simulink model "opti_debug"  (R2023a)
settings: Solver=FixedStepAuto  StartTime=0.0  StopTime=mdl.rt  RelTol=1e-3
values from neighbouring files (symbols this model uses):
  archived_Eul_XYZ = rst_Eul_XYZ.signals.values    [s4_run.m]    (also in step4_run_v1.m)
  archived_p_raw = rst_p_raw.signals.values    [s4_run.m]    (also in step4_run_v1.m)
  ctr = make_ext_tor_observer(rsim, mdl, ctr)    [s1_setup.m]    (also in setup_controller_with_functions.m = make_controller(); step1_setup.m; step1_setup_v1.m)
  ctr2 = ctr    [s1_setup.m]    (also in step1_setup.m; step1_setup_v1.m)
  lut = gen_lut    [s1_setup.m]    (also in thrust2voltage_lut_20230809.mat = ; thrust2voltage_lut_20230829.mat = )
  mdl = make_model(mdl,rsim)    [s1_setup.m]    (also in setup_controller_with_functions.m = make_model(flight_time); step1_setup.m; step1_setup_v1.m = make_model(flight_time,rsim))
  rbt = make_robot    [s1_setup.m]    (also in setup_controller_with_functions.m = make_robot(); step1_setup.m; step1_setup_v1.m)
  rbt2 = rbt    [s1_setup.m]    (also in step1_setup.m; step1_setup_v1.m)
  rsim = make_robot_simulation()    [setup_controller_with_functions.m]    (also in step1_setup_v1.m = make_simulation(rbt,mdl,rsim))
  sen = make_sensor(mdl,rsim)    [s1_setup.m]
  som = make_somersault(mdl, rsim)    [s1_setup.m]    (also in step1_setup.m)
  Time = logsout.LiveStreamSignals.getElement('voltage').Values.Time    [old_step3_run_controller_v3.m]    (also in post_identify_actuation_response.m = yout(:,1); post_thrust_torque_coefficients.m = yout(:,1))
  traj = make_trajectory(ctr, mdl, rsim)    [s1_setup.m]    (also in step1_setup.m)
undefined symbols (not defined in the file or in its folder): DiscIntNeverNeededParam, Discrete, Standard_Devices, UDP_Protocol
libraries: simulink x27, dspfdesign x12, robotcorelib x7, sldrtlib x7, slrealtimeloglib x1, shared6dof x1, dspsrcs4 x1, uavutilslib x1, ctrlSharedLib x1, dspmathops x1
(part 3 of 4)

== system opti_debug/State filters/Acc through derivative/Subsystem1 ==
  p_dot : Inport
  data ready : Inport  Port=2
  Add1 : Sum  Inputs=+-
  Add2 : Sum  Inputs=+-
  Add3 : Sum  Commented=on  Inputs=+-
  Add4 : Sum  Inputs=+-
  Delay : Delay  Commented=on  DelayLength=1  InitialCondition=zeros(3,1)
  Delay1 : Delay  DelayLength=1  InitialCondition=zeros(3,1)
  Digital Filter Design2 : dspfdesign/Digital Filter Design  Commented=on  mwdsp_browser_bugfix_var=off
  Digital Clock : DigitalClock  SampleTime=mdl.T_high
  Gain : Gain  Commented=on  Gain=mdl.f_high
  Gain1 : Gain  Gain=mdl.f_high
  If : If  IfExpression=u1 == 0
  If Action Subsystem : Subsystem  TreatAsAtomicUnit=on
  If Action Subsystem1 : Subsystem  TreatAsAtomicUnit=on
  Merge : Merge
  Scope : Scope  Commented=on  NumInputPorts=2
  Triggered Subsystem : Subsystem  TreatAsAtomicUnit=on
  p_dotdot : Outport
  wires:
  data ready/1 -> Triggered Subsystem/Trigger
  Triggered Subsystem/1(Out1) -> Add1/1
  Triggered Subsystem/2(Output) -> Add1/2
  Triggered Subsystem/3(Output1) -> Add2/1
  Triggered Subsystem/4(Output2) -> Add2/2
  Add1/1 -> If Action Subsystem/1(In1)
  Add2/1 -> If Action Subsystem/2(In2), If/1
  If/2 -> If Action Subsystem/Action
  If/1 -> If Action Subsystem1/Action
  If Action Subsystem1/1(Out1) -> Merge/2
  If Action Subsystem/1(Out1) -> Merge/1
  Digital Clock/1 -> Triggered Subsystem/2(In2)
  Digital Filter Design2/1 -> Delay/1, Add3/1  "p_dot_filtered"
  Delay/1 -> Add3/2
  Add3/1 -> Gain/1
  Gain/1 -> Scope/2
  Add4/1 -> Gain1/1
  Delay1/1 -> Add4/2
  p_dot/1 -> Delay1/1, Add4/1, Digital Filter Design2/1, Triggered Subsystem/1(In1)  "p_dot_filtered"
  Gain1/1 -> p_dotdot/1, Scope/1

== system opti_debug/State filters/IMU orientation/Subsystem2 ==
  euler_angles : Inport
  Add1 : Sum  Commented=on  Inputs=+-
  Add2 : Sum  Commented=on  Inputs=+-
  Digital Clock : DigitalClock  Commented=on  SampleTime=1/10000
  If : If  Commented=on  IfExpression=u1 == 0
  If Action Subsystem : Subsystem  Commented=on  TreatAsAtomicUnit=on
  If Action Subsystem1 : Subsystem  Commented=on  TreatAsAtomicUnit=on
  MATLAB Function : MATLAB Function  TreatAsAtomicUnit=on
  Merge : Merge  Commented=on
  Rotation Matrix : MATLAB Function  TreatAsAtomicUnit=on
  Rotation Matrix3 : MATLAB Function  TreatAsAtomicUnit=on
  Triggered Subsystem : Subsystem  Commented=on  TreatAsAtomicUnit=on
  Omega : Outport
  wires:
  Triggered Subsystem/1(Out1) -> Add1/1
  Triggered Subsystem/3(Output1) -> Add2/1
  Triggered Subsystem/4(Output2) -> Add2/2
  If Action Subsystem1/1(Out1) -> Merge/2
  If Action Subsystem/1(Out1) -> Merge/1
  Triggered Subsystem/2(Output) -> Add1/2
  Digital Clock/1 -> Triggered Subsystem/2(In2)
  Add2/1 -> If Action Subsystem/2(In2), If/1
  If/2 -> If Action Subsystem/Action
  If/1 -> If Action Subsystem1/Action
  Add1/1 -> If Action Subsystem/1(In1)
  euler_angles/1 -> MATLAB Function/1(Eul_in), Rotation Matrix/1(euler_angles)
  Rotation Matrix/1(R) -> Rotation Matrix3/1(R)
  Rotation Matrix3/1(w) -> Omega/1  "Vicon_omega"
  MATLAB Function/1(R_dot) -> Rotation Matrix3/2(Rdot)

== system opti_debug/State filters/Velocity through derivative/Subsystem4 ==
  In1 : Inport
  data ready : Inport  Port=2
  Add1 : Sum  Inputs=+-
  Add2 : Sum  Inputs=+-
  Digital Filter Design1 : dspfdesign/Digital Filter Design  mwdsp_browser_bugfix_var=off
  Digital Filter Design2 : dspfdesign/Digital Filter Design  Commented=on  mwdsp_browser_bugfix_var=off
  Digital Clock : DigitalClock  SampleTime=mdl.T_high
  If : If  IfExpression=u1 == 0
  If Action Subsystem : Subsystem  TreatAsAtomicUnit=on
  If Action Subsystem1 : Subsystem  TreatAsAtomicUnit=on
  Merge : Merge
  Scope : Scope  Commented=on  NumInputPorts=2
  Triggered Subsystem : Subsystem  TreatAsAtomicUnit=on
  p dot : Outport
  wires:
  In1/1 -> Triggered Subsystem/1(In1)
  data ready/1 -> Triggered Subsystem/Trigger
  Triggered Subsystem/1(Out1) -> Add1/1
  Triggered Subsystem/2(Output) -> Add1/2
  Triggered Subsystem/3(Output1) -> Add2/1
  Triggered Subsystem/4(Output2) -> Add2/2
  Add1/1 -> If Action Subsystem/1(In1)
  Add2/1 -> If Action Subsystem/2(In2), If/1
  If/2 -> If Action Subsystem/Action
  If/1 -> If Action Subsystem1/Action
  If Action Subsystem1/1(Out1) -> Merge/2
  If Action Subsystem/1(Out1) -> Merge/1
  Merge/1 -> Digital Filter Design1/1, Scope/1
  Digital Clock/1 -> Triggered Subsystem/2(In2)
  Digital Filter Design1/1 -> Scope/2, p dot/1  "p_dot_filtered"

== system opti_debug/State filters/Vicon orientation/Subsystem5 ==
  euler_angles : Inport
  data ready : Inport  Port=2
  Add1 : Sum  Inputs=+-
  Add2 : Sum  Inputs=+-
  Add3 : Sum  Inputs=+-
  Constant : Constant  Value=rsim.en
  Delay : Delay  DelayLength=1  InitialCondition=zeros(9,1)
  Digital Clock : DigitalClock  SampleTime=1/10000
  Gain : Gain  Gain=400
  If : If  IfExpression=u1 == 0
  If Action Subsystem : Subsystem  TreatAsAtomicUnit=on
  If Action Subsystem1 : Subsystem  TreatAsAtomicUnit=on
  Merge : Merge
  Rotation Matrix : MATLAB Function  TreatAsAtomicUnit=on
  Rotation Matrix2 : MATLAB Function  TreatAsAtomicUnit=on
  Rotation Matrix3 : MATLAB Function  TreatAsAtomicUnit=on
  Switch1 : Switch  Criteria=u2 > Threshold  SaturateOnIntegerOverflow=off  InputSameDT=off
  Switch2 : Switch  Criteria=u2 > Threshold  SaturateOnIntegerOverflow=off  InputSameDT=off
  Triggered Subsystem : Subsystem  TreatAsAtomicUnit=on
  R : Outport
  Rdot : Outport  Port=2
  Omega : Outport  Port=3
  wires:
  Triggered Subsystem/1(Out1) -> Add1/1
  Triggered Subsystem/3(Output1) -> Add2/1
  Triggered Subsystem/4(Output2) -> Add2/2
  If Action Subsystem1/1(Out1) -> Merge/2
  If Action Subsystem/1(Out1) -> Merge/1
  Triggered Subsystem/2(Output) -> Add1/2
  Digital Clock/1 -> Triggered Subsystem/2(In2)
  data ready/1 -> Triggered Subsystem/Trigger
  Add2/1 -> If Action Subsystem/2(In2), If/1
  If/2 -> If Action Subsystem/Action
  If/1 -> If Action Subsystem1/Action
  Add1/1 -> If Action Subsystem/1(In1)
  euler_angles/1 -> Rotation Matrix/1(euler_angles)
  Rotation Matrix/1(R) -> Triggered Subsystem/1(R), R/1, Rotation Matrix3/1(R), Rotation Matrix2/1(R), Delay/1, Add3/1
  Delay/1 -> Add3/2
  Add3/1 -> Gain/1
  Constant/1 -> Switch2/2, Switch1/2
  Gain/1 -> Switch2/1, Rotation Matrix2/2(Rdot)
  Rotation Matrix2/1(w) -> Switch1/1  "sim_omega"
  Merge/1 -> Switch2/3, Rotation Matrix3/2(Rdot)
  Rotation Matrix3/1(w) -> Switch1/3  "Vicon_omega"
  Switch1/1 -> Omega/1  "p_raw"
  Switch2/1 -> Rdot/1  "p_raw"

== system opti_debug/Control scheme/attitude and thrust controller/Yaw Controller/start ramp ==
  0.8 : Constant  Value=0.01
  2 : Constant  Value=mdl.i_delay
  Add1 : Sum
  Add2 : Sum  Inputs=+-
  Compare To Zero : simulink/Logic and Bit Operations/Compare To Zero  relop=>  OutDataTypeStr=uint8  ZeroCross=off
  Data Type Conversion : DataTypeConversion  SaturateOnIntegerOverflow=off  RndMeth=Floor
  constant : Constant
  counter : DiscreteIntegrator  gainval=1  SampleTime=-1  UpperSaturationLimit=1  LowerSaturationLimit=0  ICPrevOutput=DiscIntNeverNeededParam  ICPrevScaledInput=DiscIntNeverNeededParam
  saturation ramp : DiscreteIntegrator  gainval=5  SampleTime=-1  LimitOutput=on  UpperSaturationLimit=1  LowerSaturationLimit=-1  ICPrevOutput=DiscIntNeverNeededParam  ICPrevScaledInput=DiscIntNeverNeededParam
  Out1 : Outport
  wires:
  constant/1 -> counter/1
  2/1 -> Add1/1
  0.8/1 -> Add1/2
  counter/1 -> Add2/1
  Add1/1 -> Add2/2
  Add2/1 -> Compare To Zero/1
  Compare To Zero/1 -> Data Type Conversion/1
  saturation ramp/1 -> Out1/1
  Data Type Conversion/1 -> saturation ramp/1

== system opti_debug/Control scheme/observer/Rotaion/filtered derivative ==
  In1 : Inport
  att_s : Gain  Gain=mdl.f1
  filtered derivative : simulink/Discrete/Transfer Fcn Lead or Lag  PoleZ=mdl.zf1  ZeroZ=1  ICPrevOutput=0.0  ICPrevInput=0.0  DoSatur=off
  low pass3 : DiscreteTransferFcn  Numerator=mdl.vlp.n  Denominator=mdl.vlp.d
  Out1 : Outport
  wires:
  filtered derivative/1 -> low pass3/1
  att_s/1 -> filtered derivative/1
  In1/1 -> att_s/1
  low pass3/1 -> Out1/1

== system opti_debug/Control scheme/observer/lateral observer/saturation ==
  In1 : Inport
  MinMax2 : MinMax  Inputs=2
  MinMax3 : MinMax  Function=max  Inputs=2
  lw1 : Constant  Value=-mdl.fd_lim
  up1 : Constant  Value=mdl.fd_lim
  Out1 : Outport
  wires:
  In1/1 -> MinMax2/2
  up1/1 -> MinMax2/1
  lw1/1 -> MinMax3/1
  MinMax2/1 -> MinMax3/2
  MinMax3/1 -> Out1/1

== system opti_debug/Signal generater/signal generator1/Bias_Signal/AveragedBias ==
  note: To avoid having signal "jump",
      | we want SMOOTH transitions
      | in frequency (i.e., a weighted sum
      | of current freq and freq some delta t ago)
  note: time constant = 0.002sec
  In1 : Inport
  Discrete Transfer Fcn : DiscreteTransferFcn  Commented=through  Numerator=[0.05]  Denominator=[1 -.95]
  Out1 : Outport
  wires:
  In1/1 -> Discrete Transfer Fcn/1
  Discrete Transfer Fcn/1 -> Out1/1

== system opti_debug/Signal generater/signal generator1/Bias_Signal/SIgnalForRamp_binary ==
  note: Should output 1 or -1,
      | so signal ramps UP to 1
      | or DOWN to 0.
  In1 : Inport
  Add : Sum  Inputs=+-
  Compare To Zero : simulink/Logic and Bit Operations/Compare To Zero  relop=>  OutDataTypeStr=uint8  ZeroCross=off
  Constant : Constant
  Data Type Conversion : DataTypeConversion  OutDataTypeStr=double  SaturateOnIntegerOverflow=off  RndMeth=Floor
  Gain : Gain  Gain=2
  Out1 : Outport
  wires:
  In1/1 -> Compare To Zero/1
  Compare To Zero/1 -> Data Type Conversion/1
  Gain/1 -> Add/1
  Constant/1 -> Add/2
  Add/1 -> Out1/1
  Data Type Conversion/1 -> Gain/1

== system opti_debug/Signal generater/signal generator1/Drive_Signal1/AveragedAmp_filtered ==
  note: To avoid having signal "jump",
      | we want SMOOTH transitions
      | in frequency (i.e., a weighted sum
      | of current freq and freq some delta t ago)
  note: time constant 0.002sec
      | for 10kHz samping
  In1 : Inport
  Discrete Transfer Fcn : DiscreteTransferFcn  Commented=through  Numerator=[0.05]  Denominator=[1 -.95]
  Out1 : Outport
  wires:
  In1/1 -> Discrete Transfer Fcn/1
  Discrete Transfer Fcn/1 -> Out1/1

== system opti_debug/Signal generater/signal generator1/Drive_Signal1/AveragedOffset_filtered ==
  note: To avoid having signal "jump",
      | we want SMOOTH transitions
      | in frequency (i.e., a weighted sum
      | of current freq and freq some delta t ago)
  note: c
  note: time constant 0.02sec
      | for 10kHz samping
  In1 : Inport
  Discrete Transfer Fcn : DiscreteTransferFcn  Commented=through  Numerator=[0.05]  Denominator=[1 -.95]
  Out1 : Outport
  wires:
  In1/1 -> Discrete Transfer Fcn/1
  Discrete Transfer Fcn/1 -> Out1/1

== system opti_debug/Signal generater/signal generator1/Drive_Signal1/AveragedTau_filtered ==
  note: To avoid having signal "jump",
      | we want SMOOTH transitions
      | in frequency (i.e., a weighted sum
      | of current freq and freq some delta t ago)
  note: time constant 0.002sec
      | for 10kHz samping
  In1 : Inport
  Discrete Transfer Fcn : DiscreteTransferFcn  Numerator=[0.05]  Denominator=[1, -0.95]
  Out1 : Outport
  wires:
  In1/1 -> Discrete Transfer Fcn/1
  Discrete Transfer Fcn/1 -> Out1/1

== system opti_debug/Signal generater/signal generator1/Drive_Signal1/SignalForRamp_binary ==
  note: Should output 1 or -1,
      | so signal ramps UP to 1
      | or DOWN to 0.
  In1 : Inport
  Add : Sum  Inputs=+-
  Compare To Zero : simulink/Logic and Bit Operations/Compare To Zero  relop=>  OutDataTypeStr=uint8  ZeroCross=off
  Constant : Constant
  Data Type Conversion : DataTypeConversion  OutDataTypeStr=double  SaturateOnIntegerOverflow=off  RndMeth=Floor
  Gain : Gain  Gain=2
  Out1 : Outport
  wires:
  In1/1 -> Compare To Zero/1
  Compare To Zero/1 -> Data Type Conversion/1
  Gain/1 -> Add/1
  Constant/1 -> Add/2
  Add/1 -> Out1/1
  Data Type Conversion/1 -> Gain/1

== system opti_debug/Signal generater/signal generator1/Drive_Signal1/SignalForSin_binary ==
  note: We want this to stay "high" for 1
      | second after the actual "enable"
      | is turned off...
  In1 : Inport
  Compare To Zero : simulink/Logic and Bit Operations/Compare To Zero  relop=>  OutDataTypeStr=uint8  ZeroCross=off
  Data Type Conversion : DataTypeConversion  OutDataTypeStr=double  SaturateOnIntegerOverflow=off  RndMeth=Floor
  Out1 : Outport
  wires:
  In1/1 -> Compare To Zero/1
  Compare To Zero/1 -> Data Type Conversion/1
  Data Type Conversion/1 -> Out1/1

== system opti_debug/Signal generater/signal generator1/Drive_Signal1/Subsystem ==
  note: positive value pushes the left wing forward
  split cycle mu : Inport
  In2 : Inport  Port=2
  1-mu : Sum  Inputs=+-
  2f : Gain  Gain=2
  2nd harmonic : Trigonometry  OutputSignalType=real
  2pi : Gain  Gain=2*pi
  Abs1 : Abs  SaturateOnIntegerOverflow=off
  Add : Sum
  Constant : Constant
  combined sines : Sum
  deg to rad : Gain  Gain=pi/180
  f : Gain  Gain=-1
  first harmonic : Trigonometry  OutputSignalType=real
  omega*t : DiscreteIntegrator  SampleTime=-1  ICPrevOutput=DiscIntNeverNeededParam  ICPrevScaledInput=DiscIntNeverNeededParam
  phase offset : Constant  Value=0
  signal with gain1 : Product  RndMeth=Zero
  signal with gain2 : Product  RndMeth=Zero
  split cycle signal : Outport
  wires:
  2f/1 -> 2nd harmonic/1
  first harmonic/1 -> signal with gain1/2
  Constant/1 -> 1-mu/1
  split cycle mu/1 -> f/1, Abs1/1
  1-mu/1 -> signal with gain1/1
  2nd harmonic/1 -> signal with gain2/2
  signal with gain1/1 -> combined sines/1
  signal with gain2/1 -> combined sines/2
  combined sines/1 -> split cycle signal/1
  f/1 -> signal with gain2/1
  Abs1/1 -> 1-mu/2
  In2/1 -> 2pi/1
  2pi/1 -> omega*t/1
  omega*t/1 -> Add/2
  Add/1 -> first harmonic/1, 2f/1
  phase offset/1 -> deg to rad/1
  deg to rad/1 -> Add/1

== system opti_debug/Signal generater/signal generator1/Drive_Signal2/AveragedAmp_filtered ==
  note: To avoid having signal "jump",
      | we want SMOOTH transitions
      | in frequency (i.e., a weighted sum
      | of current freq and freq some delta t ago)
  note: time constant 0.002sec
      | for 10kHz samping
  In1 : Inport
  Discrete Transfer Fcn : DiscreteTransferFcn  Numerator=[0.05]  Denominator=[1 -.95]
  Out1 : Outport
  wires:
  In1/1 -> Discrete Transfer Fcn/1
  Discrete Transfer Fcn/1 -> Out1/1

== system opti_debug/Signal generater/signal generator1/Drive_Signal2/AveragedOffset_filtered ==
  note: To avoid having signal "jump",
      | we want SMOOTH transitions
      | in frequency (i.e., a weighted sum
      | of current freq and freq some delta t ago)
  note: c
  note: time constant 0.02sec
      | for 10kHz samping
  In1 : Inport
  Discrete Transfer Fcn : DiscreteTransferFcn  Numerator=[0.05]  Denominator=[1 -.95]
  Out1 : Outport
  wires:
  In1/1 -> Discrete Transfer Fcn/1
  Discrete Transfer Fcn/1 -> Out1/1

== system opti_debug/Signal generater/signal generator1/Drive_Signal2/AveragedTau_filtered ==
  note: To avoid having signal "jump",
      | we want SMOOTH transitions
      | in frequency (i.e., a weighted sum
      | of current freq and freq some delta t ago)
  note: time constant 0.002sec
      | for 10kHz samping
  In1 : Inport
  Discrete Transfer Fcn : DiscreteTransferFcn  Numerator=[0.05]  Denominator=[1, -0.95]
  Out1 : Outport
  wires:
  In1/1 -> Discrete Transfer Fcn/1
  Discrete Transfer Fcn/1 -> Out1/1

== system opti_debug/Signal generater/signal generator1/Drive_Signal2/SignalForRamp_binary ==
  note: Should output 1 or -1,
      | so signal ramps UP to 1
      | or DOWN to 0.
  In1 : Inport
  Add : Sum  Inputs=+-
  Compare To Zero : simulink/Logic and Bit Operations/Compare To Zero  relop=>  OutDataTypeStr=uint8  ZeroCross=off
  Constant : Constant
  Data Type Conversion : DataTypeConversion  OutDataTypeStr=double  SaturateOnIntegerOverflow=off  RndMeth=Floor
  Gain : Gain  Gain=2
  Out1 : Outport
  wires:
  In1/1 -> Compare To Zero/1
  Compare To Zero/1 -> Data Type Conversion/1
  Gain/1 -> Add/1
  Constant/1 -> Add/2
  Add/1 -> Out1/1
  Data Type Conversion/1 -> Gain/1

== system opti_debug/Signal generater/signal generator1/Drive_Signal2/SignalForSin_binary ==
  note: We want this to stay "high" for 1
      | second after the actual "enable"
      | is turned off...
  In1 : Inport
  Compare To Zero : simulink/Logic and Bit Operations/Compare To Zero  relop=>  OutDataTypeStr=uint8  ZeroCross=off
  Data Type Conversion : DataTypeConversion  OutDataTypeStr=double  SaturateOnIntegerOverflow=off  RndMeth=Floor
  Out1 : Outport
  wires:
  In1/1 -> Compare To Zero/1
  Compare To Zero/1 -> Data Type Conversion/1
  Data Type Conversion/1 -> Out1/1

== system opti_debug/Signal generater/signal generator1/Drive_Signal2/Subsystem ==
  note: positive value pushes the left wing forward
  split cycle mu : Inport
  In2 : Inport  Port=2
  1-mu : Sum  Inputs=+-
  2f : Gain  Gain=2
  2nd harmonic : Trigonometry  OutputSignalType=real
  2pi : Gain  Gain=2*pi
  Abs1 : Abs  SaturateOnIntegerOverflow=off
  Add : Sum
  Constant : Constant
  combined sines : Sum
  deg to rad : Gain  Gain=pi/180
  f : Gain  Gain=-1
  first harmonic : Trigonometry  OutputSignalType=real
  omega*t : DiscreteIntegrator  SampleTime=-1  ICPrevOutput=DiscIntNeverNeededParam  ICPrevScaledInput=DiscIntNeverNeededParam
  phase offset : Constant  Value=0
  signal with gain1 : Product  RndMeth=Zero
  signal with gain2 : Product  RndMeth=Zero
  split cycle signal : Outport
  wires:
  2f/1 -> 2nd harmonic/1
  first harmonic/1 -> signal with gain1/2
  Constant/1 -> 1-mu/1
  split cycle mu/1 -> f/1, Abs1/1
  1-mu/1 -> signal with gain1/1
  2nd harmonic/1 -> signal with gain2/2
  signal with gain1/1 -> combined sines/1
  signal with gain2/1 -> combined sines/2
  combined sines/1 -> split cycle signal/1
  f/1 -> signal with gain2/1
  Abs1/1 -> 1-mu/2
  In2/1 -> 2pi/1
  2pi/1 -> omega*t/1
  omega*t/1 -> Add/2
  Add/1 -> first harmonic/1, 2f/1
  phase offset/1 -> deg to rad/1
  deg to rad/1 -> Add/1

== system opti_debug/Signal generater/signal generator1/Drive_Signal3/AveragedAmp_filtered ==
  note: To avoid having signal "jump",
      | we want SMOOTH transitions
      | in frequency (i.e., a weighted sum
      | of current freq and freq some delta t ago)
  note: time constant 0.002sec
      | for 10kHz samping
  In1 : Inport
  Discrete Transfer Fcn : DiscreteTransferFcn  Numerator=[0.05]  Denominator=[1 -.95]
  Out1 : Outport
  wires:
  In1/1 -> Discrete Transfer Fcn/1
  Discrete Transfer Fcn/1 -> Out1/1

== system opti_debug/Signal generater/signal generator1/Drive_Signal3/AveragedOffset_filtered ==
  note: To avoid having signal "jump",
      | we want SMOOTH transitions
      | in frequency (i.e., a weighted sum
      | of current freq and freq some delta t ago)
  note: c
  note: time constant 0.02sec
      | for 10kHz samping
  In1 : Inport
  Discrete Transfer Fcn : DiscreteTransferFcn  Numerator=[0.05]  Denominator=[1 -.95]
  Out1 : Outport
  wires:
  In1/1 -> Discrete Transfer Fcn/1
  Discrete Transfer Fcn/1 -> Out1/1

== system opti_debug/Signal generater/signal generator1/Drive_Signal3/AveragedTau_filtered ==
  note: To avoid having signal "jump",
      | we want SMOOTH transitions
      | in frequency (i.e., a weighted sum
      | of current freq and freq some delta t ago)
  note: time constant 0.002sec
      | for 10kHz samping
  In1 : Inport
  Discrete Transfer Fcn : DiscreteTransferFcn  Numerator=[0.05]  Denominator=[1 -.95]
  Out1 : Outport
  wires:
  In1/1 -> Discrete Transfer Fcn/1
  Discrete Transfer Fcn/1 -> Out1/1

== system opti_debug/Signal generater/signal generator1/Drive_Signal3/SignalForRamp_binary ==
  note: Should output 1 or -1,
      | so signal ramps UP to 1
      | or DOWN to 0.
  In1 : Inport
  Add : Sum  Inputs=+-
  Compare To Zero : simulink/Logic and Bit Operations/Compare To Zero  relop=>  OutDataTypeStr=uint8  ZeroCross=off
  Constant : Constant
  Data Type Conversion : DataTypeConversion  OutDataTypeStr=double  SaturateOnIntegerOverflow=off  RndMeth=Floor
  Gain : Gain  Gain=2
  Out1 : Outport
  wires:
  In1/1 -> Compare To Zero/1
  Compare To Zero/1 -> Data Type Conversion/1
  Gain/1 -> Add/1
  Constant/1 -> Add/2
  Add/1 -> Out1/1
  Data Type Conversion/1 -> Gain/1

== system opti_debug/Signal generater/signal generator1/Drive_Signal3/SignalForSin_binary ==
  note: We want this to stay "high" for 1
      | second after the actual "enable"
      | is turned off...
  In1 : Inport
  Compare To Zero : simulink/Logic and Bit Operations/Compare To Zero  relop=>  OutDataTypeStr=uint8  ZeroCross=off
  Data Type Conversion : DataTypeConversion  OutDataTypeStr=double  SaturateOnIntegerOverflow=off  RndMeth=Floor
  Out1 : Outport
  wires:
  In1/1 -> Compare To Zero/1
  Compare To Zero/1 -> Data Type Conversion/1
  Data Type Conversion/1 -> Out1/1

== system opti_debug/Signal generater/signal generator1/Drive_Signal3/Subsystem ==
  split cycle mu : Inport
  In2 : Inport  Port=2
  1-mu : Sum  Inputs=+-
  2f : Gain  Gain=2
  2nd harmonic : Trigonometry  OutputSignalType=real
  2pi : Gain  Gain=2*pi
  Abs1 : Abs  SaturateOnIntegerOverflow=off
  Constant : Constant
  SmoothClock : DiscreteIntegrator  SampleTime=-1  ICPrevOutput=DiscIntNeverNeededParam  ICPrevScaledInput=DiscIntNeverNeededParam
  combined sines : Sum
  f : Gain
  first harmonic : Trigonometry  OutputSignalType=real
  signal with gain1 : Product  RndMeth=Zero
  signal with gain2 : Product  RndMeth=Zero
  split cycle signal : Outport
  wires:
  SmoothClock/1 -> first harmonic/1, 2f/1
  2f/1 -> 2nd harmonic/1
  2pi/1 -> SmoothClock/1
  first harmonic/1 -> signal with gain1/2
  Constant/1 -> 1-mu/1
  split cycle mu/1 -> f/1, Abs1/1
  1-mu/1 -> signal with gain1/1
  2nd harmonic/1 -> signal with gain2/2
  signal with gain1/1 -> combined sines/1
  signal with gain2/1 -> combined sines/2
  combined sines/1 -> split cycle signal/1
  In2/1 -> 2pi/1
  f/1 -> signal with gain2/1
  Abs1/1 -> 1-mu/2

== system opti_debug/Signal generater/signal generator1/Drive_Signal4/AveragedAmp_filtered ==
  note: To avoid having signal "jump",
      | we want SMOOTH transitions
      | in frequency (i.e., a weighted sum
      | of current freq and freq some delta t ago)
  note: time constant 0.002sec
      | for 10kHz samping
  In1 : Inport
  Discrete Transfer Fcn : DiscreteTransferFcn  Commented=through  Numerator=[0.05]  Denominator=[1 -.95]
  Out1 : Outport
  wires:
  In1/1 -> Discrete Transfer Fcn/1
  Discrete Transfer Fcn/1 -> Out1/1

== system opti_debug/Signal generater/signal generator1/Drive_Signal4/AveragedOffset_filtered ==
  note: To avoid having signal "jump",
      | we want SMOOTH transitions
      | in frequency (i.e., a weighted sum
      | of current freq and freq some delta t ago)
  note: c
  note: time constant 0.02sec
      | for 10kHz samping
  In1 : Inport
  Discrete Transfer Fcn : DiscreteTransferFcn  Commented=through  Numerator=[0.05]  Denominator=[1 -.95]
  Out1 : Outport
  wires:
  In1/1 -> Discrete Transfer Fcn/1
  Discrete Transfer Fcn/1 -> Out1/1

== system opti_debug/Signal generater/signal generator1/Drive_Signal4/AveragedTau_filtered ==
  note: To avoid having signal "jump",
      | we want SMOOTH transitions
      | in frequency (i.e., a weighted sum
      | of current freq and freq some delta t ago)
  note: time constant 0.002sec
      | for 10kHz samping
  In1 : Inport
  Discrete Transfer Fcn : DiscreteTransferFcn  Numerator=[0.05]  Denominator=[1, -0.95]
  Out1 : Outport
  wires:
  In1/1 -> Discrete Transfer Fcn/1
  Discrete Transfer Fcn/1 -> Out1/1

== system opti_debug/Signal generater/signal generator1/Drive_Signal4/SignalForRamp_binary ==
  note: Should output 1 or -1,
      | so signal ramps UP to 1
      | or DOWN to 0.
  In1 : Inport
  Add : Sum  Inputs=+-
  Compare To Zero : simulink/Logic and Bit Operations/Compare To Zero  relop=>  OutDataTypeStr=uint8  ZeroCross=off
  Constant : Constant
  Data Type Conversion : DataTypeConversion  OutDataTypeStr=double  SaturateOnIntegerOverflow=off  RndMeth=Floor
  Gain : Gain  Gain=2
  Out1 : Outport
  wires:
  In1/1 -> Compare To Zero/1
  Compare To Zero/1 -> Data Type Conversion/1
  Gain/1 -> Add/1
  Constant/1 -> Add/2
  Add/1 -> Out1/1
  Data Type Conversion/1 -> Gain/1

== system opti_debug/Signal generater/signal generator1/Drive_Signal4/SignalForSin_binary ==
  note: We want this to stay "high" for 1
      | second after the actual "enable"
      | is turned off...
  In1 : Inport
  Compare To Zero : simulink/Logic and Bit Operations/Compare To Zero  relop=>  OutDataTypeStr=uint8  ZeroCross=off
  Data Type Conversion : DataTypeConversion  OutDataTypeStr=double  SaturateOnIntegerOverflow=off  RndMeth=Floor
  Out1 : Outport
  wires:
  In1/1 -> Compare To Zero/1
  Compare To Zero/1 -> Data Type Conversion/1
  Data Type Conversion/1 -> Out1/1

== system opti_debug/Signal generater/signal generator1/Drive_Signal4/Subsystem ==
  note: positive value pushes the left wing forward
  split cycle mu : Inport
  In2 : Inport  Port=2
  1-mu : Sum  Inputs=+-
  2f : Gain  Gain=2
  2nd harmonic : Trigonometry  OutputSignalType=real
  2pi : Gain  Gain=2*pi
  Abs1 : Abs  SaturateOnIntegerOverflow=off
  Add : Sum
  Constant : Constant
  combined sines : Sum
  deg to rad : Gain  Gain=pi/180
  f : Gain  Gain=-1
  first harmonic : Trigonometry  OutputSignalType=real
  omega*t : DiscreteIntegrator  SampleTime=-1  ICPrevOutput=DiscIntNeverNeededParam  ICPrevScaledInput=DiscIntNeverNeededParam
  phase offset : Constant  Value=0
  signal with gain1 : Product  RndMeth=Zero
  signal with gain2 : Product  RndMeth=Zero
  split cycle signal : Outport
  wires:
  2f/1 -> 2nd harmonic/1
  first harmonic/1 -> signal with gain1/2
  Constant/1 -> 1-mu/1
  split cycle mu/1 -> f/1, Abs1/1
  1-mu/1 -> signal with gain1/1
  2nd harmonic/1 -> signal with gain2/2
  signal with gain1/1 -> combined sines/1
  signal with gain2/1 -> combined sines/2
  combined sines/1 -> split cycle signal/1
  f/1 -> signal with gain2/1
  Abs1/1 -> 1-mu/2
  In2/1 -> 2pi/1
  2pi/1 -> omega*t/1
  omega*t/1 -> Add/2
  Add/1 -> first harmonic/1, 2f/1
  phase offset/1 -> deg to rad/1
  deg to rad/1 -> Add/1

== system opti_debug/Signal generater/signal generator1/signal generator 1/SignalForRamp_binary ==
  note: Should output 1 or -1,
      | so signal ramps UP to 1
      | or DOWN to 0.
  EnableSignal : Inport
  Add : Sum  Inputs=+-
  Compare To Zero : simulink/Logic and Bit Operations/Compare To Zero  relop=>  OutDataTypeStr=uint8  ZeroCross=off
  Constant : Constant
  Data Type Conversion : DataTypeConversion  OutDataTypeStr=double  SaturateOnIntegerOverflow=off  RndMeth=Floor
  Gain : Gain  Gain=2
  Out1 : Outport
  wires:
  EnableSignal/1 -> Compare To Zero/1
  Compare To Zero/1 -> Data Type Conversion/1
  Gain/1 -> Add/1
  Constant/1 -> Add/2
  Add/1 -> Out1/1
  Data Type Conversion/1 -> Gain/1

== system opti_debug/Signal generater/signal generator1/signal generator 1/SignalSaturationLimit4 ==
  Max : Inport
  SignalRaw : Inport  Port=2
  MaxOf : MinMax  Function=max  Inputs=2
  MinOf : MinMax  Inputs=2
  ground : Constant
  SignalSatd : Outport
  wires:
  SignalRaw/1 -> MinOf/2
  MinOf/1 -> MaxOf/1
  MaxOf/1 -> SignalSatd/1
  Max/1 -> MinOf/1
  ground/1 -> MaxOf/2

== system opti_debug/Signal generater/signal generator1/signal generator 1/get max voltage ==
  note: time constant = 0.002sec
  QuasiEnable : Inport
  max voltage : Inport  Port=2
  Product : Product  RndMeth=Zero
  SIgnalForRamp_binary : Subsystem
  SaturatingRamp : DiscreteIntegrator  gainval=1000  SampleTime=-1  LimitOutput=on  UpperSaturationLimit=1  LowerSaturationLimit=0  ICPrevOutput=DiscIntNeverNeededParam  ICPrevScaledInput=DiscIntNeverNeededParam
  max signa; : Outport
  wires:
  Product/1 -> max signa;/1
  max voltage/1 -> Product/2
  QuasiEnable/1 -> SIgnalForRamp_binary/1(In1)
  SIgnalForRamp_binary/1(Out1) -> SaturatingRamp/1
  SaturatingRamp/1 -> Product/1

== system opti_debug/Signal generater/signal generator1/signal generator 1/original sine wave ==
  In1 : Inport
  In2 : Inport  Port=2
  new_amplitude : Inport  Port=3
  2pi : Gain  Gain=2*pi
  Add1 : Sum
  Add2 : Sum
  Gain1 : Gain  Gain=-1
  Subsystem : Subsystem
  first harmonic : Trigonometry  Operator=cos  OutputSignalType=real
  omega*t : DiscreteIntegrator  SampleTime=-1  ICPrevOutput=DiscIntNeverNeededParam  ICPrevScaledInput=DiscIntNeverNeededParam
  signal with gain1 : Product  RndMeth=Zero
  Out1 : Outport
  wires:
  signal with gain1/1 -> Add2/1
  first harmonic/1 -> Gain1/1
  omega*t/1 -> Add1/2
  Subsystem/1(output) -> signal with gain1/2, Add2/2
  In2/1 -> 2pi/1
  Add1/1 -> first harmonic/1
  Gain1/1 -> Subsystem/1(cos wave), signal with gain1/1
  2pi/1 -> omega*t/1
  In1/1 -> Add1/1
  Add2/1 -> Out1/1
  new_amplitude/1 -> Subsystem/2(new_amplitude)

== system opti_debug/Signal generater/signal generator1/signal generator 1/square root of sine wave ==
  phase : Inport
  frequency : Inport  Port=2
  half amplitude : Inport  Port=3
  2pi1 : Gain  Gain=2*pi
  Add : Sum
  Add3 : Sum
  Constant : Constant
  Gain : Gain  Gain=2
  Gain2 : Gain  Gain=1/sqrt(2)
  Sqrt : Sqrt
  Subsystem1 : Subsystem
  first harmonic1 : Trigonometry  Operator=cos  OutputSignalType=real
  omega*t1 : DiscreteIntegrator  SampleTime=-1  ICPrevOutput=DiscIntNeverNeededParam  ICPrevScaledInput=DiscIntNeverNeededParam
  signal with gain2 : Product  RndMeth=Zero
  Out1 : Outport
  wires:
  frequency/1 -> 2pi1/1
  Sqrt/1 -> Subsystem1/1(cos wave), signal with gain2/1
  Gain/1 -> Subsystem1/2(new_amplitude)
  Subsystem1/1(output) -> signal with gain2/2
  omega*t1/1 -> Add3/2
  first harmonic1/1 -> Add/1
  Constant/1 -> Add/2
  2pi1/1 -> omega*t1/1
  signal with gain2/1 -> Gain2/1
  Add/1 -> Sqrt/1
  Add3/1 -> first harmonic1/1
  half amplitude/1 -> Gain/1
  phase/1 -> Add3/1
  Gain2/1 -> Out1/1

== system opti_debug/Signal generater/signal generator1/signal generator 2/SignalForRamp_binary ==
  note: Should output 1 or -1,
      | so signal ramps UP to 1
      | or DOWN to 0.
  EnableSignal : Inport
  Add : Sum  Inputs=+-
  Compare To Zero : simulink/Logic and Bit Operations/Compare To Zero  relop=>  OutDataTypeStr=uint8  ZeroCross=off
  Constant : Constant
  Data Type Conversion : DataTypeConversion  OutDataTypeStr=double  SaturateOnIntegerOverflow=off  RndMeth=Floor
  Gain : Gain  Gain=2
  Out1 : Outport
  wires:
  EnableSignal/1 -> Compare To Zero/1
  Compare To Zero/1 -> Data Type Conversion/1
  Gain/1 -> Add/1
  Constant/1 -> Add/2
  Add/1 -> Out1/1
  Data Type Conversion/1 -> Gain/1

== system opti_debug/Signal generater/signal generator1/signal generator 2/SignalSaturationLimit4 ==
  Max : Inport
  SignalRaw : Inport  Port=2
  MaxOf : MinMax  Function=max  Inputs=2
  MinOf : MinMax  Inputs=2
  ground : Constant
  SignalSatd : Outport
  wires:
  SignalRaw/1 -> MinOf/2
  MinOf/1 -> MaxOf/1
  MaxOf/1 -> SignalSatd/1
  Max/1 -> MinOf/1
  ground/1 -> MaxOf/2

== system opti_debug/Signal generater/signal generator1/signal generator 2/Subsystem ==
  cos wave : Inport
  new_amplitude : Inport  Port=2
  Delay : Delay  DelayLength=1  InitialCondition=0
  Delay1 : Delay  InitialCondition=[0,0]
  Delay2 : Delay  DelayLength=1  InitialCondition=0
  MATLAB Function : MATLAB Function  TreatAsAtomicUnit=on  SystemSampleTime=mdl.T_high
  output : Outport
  wires:
  cos wave/1 -> Delay1/1, Delay/1, MATLAB Function/1(u1)
  MATLAB Function/1(output) -> output/1, Delay2/1
  Delay/1 -> MATLAB Function/2(u2)
  Delay2/1 -> MATLAB Function/5(old_amplitude)
  Delay1/1 -> MATLAB Function/3(u3)
  new_amplitude/1 -> MATLAB Function/4(new_amplitude)

== system opti_debug/Signal generater/signal generator1/signal generator 2/get max voltage ==
  note: time constant = 0.002sec
  QuasiEnable : Inport
  max voltage : Inport  Port=2
  Product : Product  RndMeth=Zero
  SIgnalForRamp_binary : Subsystem
  SaturatingRamp : DiscreteIntegrator  gainval=1000  SampleTime=-1  LimitOutput=on  UpperSaturationLimit=1  LowerSaturationLimit=0  ICPrevOutput=DiscIntNeverNeededParam  ICPrevScaledInput=DiscIntNeverNeededParam
  max signa; : Outport
  wires:
  Product/1 -> max signa;/1
  max voltage/1 -> Product/2
  QuasiEnable/1 -> SIgnalForRamp_binary/1(In1)
  SIgnalForRamp_binary/1(Out1) -> SaturatingRamp/1
  SaturatingRamp/1 -> Product/1

== system opti_debug/Signal generater/signal generator1/signal generator 2/square root of sine wave ==
  phase : Inport
  frequency : Inport  Port=2
  half amplitude : Inport  Port=3
  2pi1 : Gain  Gain=2*pi
  Add : Sum
  Add3 : Sum
  Constant : Constant
  Gain : Gain  Gain=2
  Gain2 : Gain  Gain=1/sqrt(2)
  Sqrt : Sqrt
  Subsystem1 : Subsystem
  first harmonic1 : Trigonometry  Operator=cos  OutputSignalType=real
  omega*t1 : DiscreteIntegrator  SampleTime=-1  ICPrevOutput=DiscIntNeverNeededParam  ICPrevScaledInput=DiscIntNeverNeededParam
  signal with gain2 : Product  RndMeth=Zero
  Out1 : Outport
  wires:
  frequency/1 -> 2pi1/1
  Sqrt/1 -> Subsystem1/1(cos wave), signal with gain2/1
  Gain/1 -> Subsystem1/2(new_amplitude)
  Subsystem1/1(output) -> signal with gain2/2
  omega*t1/1 -> Add3/2
  first harmonic1/1 -> Add/1
  Constant/1 -> Add/2
  2pi1/1 -> omega*t1/1
  signal with gain2/1 -> Gain2/1
  Add/1 -> Sqrt/1
  Add3/1 -> first harmonic1/1
  half amplitude/1 -> Gain/1
  phase/1 -> Add3/1
  Gain2/1 -> Out1/1

== system opti_debug/Signal generater/signal generator1/signal generator 3/SignalForRamp_binary ==
  note: Should output 1 or -1,
      | so signal ramps UP to 1
      | or DOWN to 0.
  EnableSignal : Inport
  Add : Sum  Inputs=+-
  Compare To Zero : simulink/Logic and Bit Operations/Compare To Zero  relop=>  OutDataTypeStr=uint8  ZeroCross=off
  Constant : Constant
  Data Type Conversion : DataTypeConversion  OutDataTypeStr=double  SaturateOnIntegerOverflow=off  RndMeth=Floor
  Gain : Gain  Gain=2
  Out1 : Outport
  wires:
  EnableSignal/1 -> Compare To Zero/1
  Compare To Zero/1 -> Data Type Conversion/1
  Gain/1 -> Add/1
  Constant/1 -> Add/2
  Add/1 -> Out1/1
  Data Type Conversion/1 -> Gain/1

== system opti_debug/Signal generater/signal generator1/signal generator 3/SignalSaturationLimit4 ==
  Max : Inport
  SignalRaw : Inport  Port=2
  MaxOf : MinMax  Function=max  Inputs=2
  MinOf : MinMax  Inputs=2
  ground : Constant
  SignalSatd : Outport
  wires:
  SignalRaw/1 -> MinOf/2
  MinOf/1 -> MaxOf/1
  MaxOf/1 -> SignalSatd/1
  Max/1 -> MinOf/1
  ground/1 -> MaxOf/2

== system opti_debug/Signal generater/signal generator1/signal generator 3/Subsystem ==
  cos wave : Inport
  new_amplitude : Inport  Port=2
  Delay : Delay  DelayLength=1  InitialCondition=0
  Delay1 : Delay  InitialCondition=[0,0]
  Delay2 : Delay  DelayLength=1  InitialCondition=0
  MATLAB Function : MATLAB Function  TreatAsAtomicUnit=on  SystemSampleTime=mdl.T_high
  output : Outport
  wires:
  cos wave/1 -> Delay1/1, Delay/1, MATLAB Function/1(u1)
  MATLAB Function/1(output) -> output/1, Delay2/1
  Delay/1 -> MATLAB Function/2(u2)
  Delay2/1 -> MATLAB Function/5(old_amplitude)
  Delay1/1 -> MATLAB Function/3(u3)
  new_amplitude/1 -> MATLAB Function/4(new_amplitude)

== system opti_debug/Signal generater/signal generator1/signal generator 3/get max voltage ==
  note: time constant = 0.002sec
  QuasiEnable : Inport
  max voltage : Inport  Port=2
  Product : Product  RndMeth=Zero
  SIgnalForRamp_binary : Subsystem
  SaturatingRamp : DiscreteIntegrator  gainval=1000  SampleTime=-1  LimitOutput=on  UpperSaturationLimit=1  LowerSaturationLimit=0  ICPrevOutput=DiscIntNeverNeededParam  ICPrevScaledInput=DiscIntNeverNeededParam
  max signa; : Outport
  wires:
  Product/1 -> max signa;/1
  max voltage/1 -> Product/2
  QuasiEnable/1 -> SIgnalForRamp_binary/1(In1)
  SIgnalForRamp_binary/1(Out1) -> SaturatingRamp/1
  SaturatingRamp/1 -> Product/1

== system opti_debug/Signal generater/signal generator1/signal generator 3/square root of sine wave ==
  phase : Inport
  frequency : Inport  Port=2
  half amplitude : Inport  Port=3
  2pi1 : Gain  Gain=2*pi
  Add : Sum
  Add3 : Sum
  Constant : Constant
  Gain : Gain  Gain=2
  Gain2 : Gain  Gain=1/sqrt(2)
  Sqrt : Sqrt
  Subsystem1 : Subsystem
  first harmonic1 : Trigonometry  Operator=cos  OutputSignalType=real
  omega*t1 : DiscreteIntegrator  SampleTime=-1  ICPrevOutput=DiscIntNeverNeededParam  ICPrevScaledInput=DiscIntNeverNeededParam
  signal with gain2 : Product  RndMeth=Zero
  Out1 : Outport
  wires:
  frequency/1 -> 2pi1/1
  Sqrt/1 -> Subsystem1/1(cos wave), signal with gain2/1
  Gain/1 -> Subsystem1/2(new_amplitude)
  Subsystem1/1(output) -> signal with gain2/2
  omega*t1/1 -> Add3/2
  first harmonic1/1 -> Add/1
  Constant/1 -> Add/2
  2pi1/1 -> omega*t1/1
  signal with gain2/1 -> Gain2/1
  Add/1 -> Sqrt/1
  Add3/1 -> first harmonic1/1
  half amplitude/1 -> Gain/1
  phase/1 -> Add3/1
  Gain2/1 -> Out1/1

== system opti_debug/Signal generater/signal generator1/signal generator 4/SignalForRamp_binary ==
  note: Should output 1 or -1,
      | so signal ramps UP to 1
      | or DOWN to 0.
  EnableSignal : Inport
  Add : Sum  Inputs=+-
  Compare To Zero : simulink/Logic and Bit Operations/Compare To Zero  relop=>  OutDataTypeStr=uint8  ZeroCross=off
  Constant : Constant
  Data Type Conversion : DataTypeConversion  OutDataTypeStr=double  SaturateOnIntegerOverflow=off  RndMeth=Floor
  Gain : Gain  Gain=2
  Out1 : Outport
  wires:
  EnableSignal/1 -> Compare To Zero/1
  Compare To Zero/1 -> Data Type Conversion/1
  Gain/1 -> Add/1
  Constant/1 -> Add/2
  Add/1 -> Out1/1
  Data Type Conversion/1 -> Gain/1

== system opti_debug/Signal generater/signal generator1/signal generator 4/SignalSaturationLimit4 ==
  Max : Inport
  SignalRaw : Inport  Port=2
  MaxOf : MinMax  Function=max  Inputs=2
  MinOf : MinMax  Inputs=2
  ground : Constant
  SignalSatd : Outport
  wires:
  SignalRaw/1 -> MinOf/2
  MinOf/1 -> MaxOf/1
  MaxOf/1 -> SignalSatd/1
  Max/1 -> MinOf/1
  ground/1 -> MaxOf/2

== system opti_debug/Signal generater/signal generator1/signal generator 4/Subsystem ==
  cos wave : Inport
  new_amplitude : Inport  Port=2
  Delay : Delay  DelayLength=1  InitialCondition=0
  Delay1 : Delay  InitialCondition=[0,0]
  Delay2 : Delay  DelayLength=1  InitialCondition=0
  MATLAB Function : MATLAB Function  TreatAsAtomicUnit=on  SystemSampleTime=mdl.T_high
  output : Outport
  wires:
  cos wave/1 -> Delay1/1, Delay/1, MATLAB Function/1(u1)
  MATLAB Function/1(output) -> output/1, Delay2/1
  Delay/1 -> MATLAB Function/2(u2)
  Delay2/1 -> MATLAB Function/5(old_amplitude)
  Delay1/1 -> MATLAB Function/3(u3)
  new_amplitude/1 -> MATLAB Function/4(new_amplitude)

== system opti_debug/Signal generater/signal generator1/signal generator 4/get max voltage ==
  note: time constant = 0.002sec
  QuasiEnable : Inport
  max voltage : Inport  Port=2
  Product : Product  RndMeth=Zero
  SIgnalForRamp_binary : Subsystem
  SaturatingRamp : DiscreteIntegrator  gainval=1000  SampleTime=-1  LimitOutput=on  UpperSaturationLimit=1  LowerSaturationLimit=0  ICPrevOutput=DiscIntNeverNeededParam  ICPrevScaledInput=DiscIntNeverNeededParam
  max signa; : Outport
  wires:
  Product/1 -> max signa;/1
  max voltage/1 -> Product/2
  QuasiEnable/1 -> SIgnalForRamp_binary/1(In1)
  SIgnalForRamp_binary/1(Out1) -> SaturatingRamp/1
  SaturatingRamp/1 -> Product/1

== system opti_debug/Signal generater/signal generator1/signal generator 4/square root of sine wave ==
  phase : Inport
  frequency : Inport  Port=2
  half amplitude : Inport  Port=3
  2pi1 : Gain  Gain=2*pi
  Add : Sum
  Add3 : Sum
  Constant : Constant
  Gain : Gain  Gain=2
  Gain2 : Gain  Gain=1/sqrt(2)
  Sqrt : Sqrt
  Subsystem1 : Subsystem
  first harmonic1 : Trigonometry  Operator=cos  OutputSignalType=real
  omega*t1 : DiscreteIntegrator  SampleTime=-1  ICPrevOutput=DiscIntNeverNeededParam  ICPrevScaledInput=DiscIntNeverNeededParam
  signal with gain2 : Product  RndMeth=Zero
  Out1 : Outport
  wires:
  frequency/1 -> 2pi1/1
  Sqrt/1 -> Subsystem1/1(cos wave), signal with gain2/1
  Gain/1 -> Subsystem1/2(new_amplitude)
  Subsystem1/1(output) -> signal with gain2/2
  omega*t1/1 -> Add3/2
  first harmonic1/1 -> Add/1
  Constant/1 -> Add/2
  2pi1/1 -> omega*t1/1
  signal with gain2/1 -> Gain2/1
  Add/1 -> Sqrt/1
  Add3/1 -> first harmonic1/1
  half amplitude/1 -> Gain/1
  phase/1 -> Add3/1
  Gain2/1 -> Out1/1

== system opti_debug/State filters/Acc through derivative/Subsystem1/If Action Subsystem ==
  In1 : Inport
  In2 : Inport  Port=2
  Action Port : ActionPort  ActionPortLabel=else
  Divide : Product  Inputs=*/
  Out1 : Outport
  wires:
  In1/1 -> Divide/1
  In2/1 -> Divide/2
  Divide/1 -> Out1/1

== system opti_debug/State filters/Acc through derivative/Subsystem1/If Action Subsystem1 ==
  Action Port : ActionPort  ActionPortLabel=if(u1 == 0)
  Constant : Constant  Value=[0;0;0]
  Out1 : Outport
  wires:
  Constant/1 -> Out1/1

== system opti_debug/State filters/Acc through derivative/Subsystem1/Triggered Subsystem ==
  In1 : Inport
  In2 : Inport  Port=2
  Trigger : TriggerPort  VariantControl=(inherit)
  Scope : Scope  Commented=on  NumInputPorts=2
  Unit Delay : UnitDelay  SampleTime=-1  HasFrameUpgradeWarning=on
  Unit Delay1 : UnitDelay  SampleTime=-1  HasFrameUpgradeWarning=on
  Out1 : Outport
  Output : Outport  Port=2
  Output1 : Outport  Port=3
  Output2 : Outport  Port=4
  wires:
  Unit Delay/1 -> Output/1
  Unit Delay1/1 -> Output2/1, Scope/2
  In1/1 -> Unit Delay/1, Out1/1
  In2/1 -> Scope/1, Output1/1, Unit Delay1/1

== system opti_debug/State filters/IMU orientation/Subsystem2/If Action Subsystem ==
  In1 : Inport
  In2 : Inport  Port=2
  Action Port : ActionPort  ActionPortLabel=else
  Divide : Product  Inputs=*/
  Out1 : Outport
  wires:
  In1/1 -> Divide/1
  In2/1 -> Divide/2
  Divide/1 -> Out1/1

== system opti_debug/State filters/IMU orientation/Subsystem2/If Action Subsystem1 ==
  Action Port : ActionPort  ActionPortLabel=if(u1 == 0)
  Constant : Constant  Value=zeros(9,1)
  Out1 : Outport
  wires:
  Constant/1 -> Out1/1

== system opti_debug/State filters/IMU orientation/Subsystem2/Triggered Subsystem ==
  R : Inport
  In2 : Inport  Port=2
  Trigger : TriggerPort  VariantControl=(inherit)
  Scope : Scope  Commented=on  NumInputPorts=2
  Unit Delay : UnitDelay  SampleTime=-1  HasFrameUpgradeWarning=on
  Unit Delay1 : UnitDelay  SampleTime=-1  HasFrameUpgradeWarning=on
  Out1 : Outport
  Output : Outport  Port=2
  Output1 : Outport  Port=3
  Output2 : Outport  Port=4
  wires:
  Unit Delay/1 -> Output/1
  Unit Delay1/1 -> Scope/2, Output2/1
  R/1 -> Unit Delay/1, Out1/1
  In2/1 -> Unit Delay1/1, Scope/1, Output1/1

== system opti_debug/State filters/Velocity through derivative/Subsystem4/If Action Subsystem ==
  In1 : Inport
  In2 : Inport  Port=2
  Action Port : ActionPort  ActionPortLabel=else
  Divide : Product  Inputs=*/
  Out1 : Outport
  wires:
  In1/1 -> Divide/1
  In2/1 -> Divide/2
  Divide/1 -> Out1/1

== system opti_debug/State filters/Velocity through derivative/Subsystem4/If Action Subsystem1 ==
  Action Port : ActionPort  ActionPortLabel=if(u1 == 0)
  Constant : Constant  Value=[0;0;0]
  Out1 : Outport
  wires:
  Constant/1 -> Out1/1

== system opti_debug/State filters/Velocity through derivative/Subsystem4/Triggered Subsystem ==
  In1 : Inport
  In2 : Inport  Port=2
  Trigger : TriggerPort  VariantControl=(inherit)
  Scope : Scope  Commented=on  NumInputPorts=2
  Unit Delay : UnitDelay  SampleTime=-1  HasFrameUpgradeWarning=on
  Unit Delay1 : UnitDelay  SampleTime=-1  HasFrameUpgradeWarning=on
  Out1 : Outport
  Output : Outport  Port=2
  Output1 : Outport  Port=3
  Output2 : Outport  Port=4
  wires:
  Unit Delay/1 -> Output/1
  Unit Delay1/1 -> Output2/1, Scope/2
  In1/1 -> Unit Delay/1, Out1/1
  In2/1 -> Scope/1, Output1/1, Unit Delay1/1

== system opti_debug/State filters/Vicon orientation/Subsystem5/If Action Subsystem ==
  In1 : Inport
  In2 : Inport  Port=2
  Action Port : ActionPort  ActionPortLabel=else
  Divide : Product  Inputs=*/
  Out1 : Outport
  wires:
  In1/1 -> Divide/1
  In2/1 -> Divide/2
  Divide/1 -> Out1/1

== system opti_debug/State filters/Vicon orientation/Subsystem5/If Action Subsystem1 ==
  Action Port : ActionPort  ActionPortLabel=if(u1 == 0)
  Constant : Constant  Value=zeros(9,1)
  Out1 : Outport
  wires:
  Constant/1 -> Out1/1

== system opti_debug/State filters/Vicon orientation/Subsystem5/Triggered Subsystem ==
  R : Inport
  In2 : Inport  Port=2
  Trigger : TriggerPort  VariantControl=(inherit)
  Scope : Scope  Commented=on  NumInputPorts=2
  Unit Delay : UnitDelay  SampleTime=-1  HasFrameUpgradeWarning=on
  Unit Delay1 : UnitDelay  SampleTime=-1  HasFrameUpgradeWarning=on
  Out1 : Outport
  Output : Outport  Port=2
  Output1 : Outport  Port=3
  Output2 : Outport  Port=4
  wires:
  Unit Delay/1 -> Output/1
  Unit Delay1/1 -> Scope/2, Output2/1
  R/1 -> Unit Delay/1, Out1/1
  In2/1 -> Unit Delay1/1, Scope/1, Output1/1

== system opti_debug/Signal generater/signal generator1/signal generator 1/get max voltage/SIgnalForRamp_binary ==
  note: Should output 1 or -1,
      | so signal ramps UP to 1
      | or DOWN to 0.
  In1 : Inport
  Add : Sum  Inputs=+-
  Compare To Zero : simulink/Logic and Bit Operations/Compare To Zero  relop=>  OutDataTypeStr=uint8  ZeroCross=off
  Constant : Constant
  Data Type Conversion : DataTypeConversion  OutDataTypeStr=double  SaturateOnIntegerOverflow=off  RndMeth=Floor
  Gain : Gain  Gain=2
  Out1 : Outport
  wires:
  In1/1 -> Compare To Zero/1
  Compare To Zero/1 -> Data Type Conversion/1
  Gain/1 -> Add/1
  Constant/1 -> Add/2
  Add/1 -> Out1/1
  Data Type Conversion/1 -> Gain/1

== system opti_debug/Signal generater/signal generator1/signal generator 1/original sine wave/Subsystem ==
  cos wave : Inport
  new_amplitude : Inport  Port=2
  Delay : Delay  DelayLength=1  InitialCondition=0
  Delay1 : Delay  InitialCondition=[0,0]
  Delay2 : Delay  DelayLength=1  InitialCondition=0
  MATLAB Function : MATLAB Function  TreatAsAtomicUnit=on  SystemSampleTime=mdl.T_high
  output : Outport
  wires:
  cos wave/1 -> Delay1/1, Delay/1, MATLAB Function/1(u1)
  MATLAB Function/1(output) -> output/1, Delay2/1
  Delay/1 -> MATLAB Function/2(u2)
  Delay2/1 -> MATLAB Function/5(old_amplitude)
  Delay1/1 -> MATLAB Function/3(u3)
  new_amplitude/1 -> MATLAB Function/4(new_amplitude)

== system opti_debug/Signal generater/signal generator1/signal generator 1/square root of sine wave/Subsystem1 ==
  cos wave : Inport
  new_amplitude : Inport  Port=2
  Delay : Delay  DelayLength=1  InitialCondition=0
  Delay1 : Delay  InitialCondition=[0,0]
  Delay2 : Delay  DelayLength=1  InitialCondition=0
  MATLAB Function : MATLAB Function  TreatAsAtomicUnit=on  SystemSampleTime=mdl.T_high
  output : Outport
  wires:
  cos wave/1 -> Delay1/1, Delay/1, MATLAB Function/1(u1)
  MATLAB Function/1(output) -> output/1, Delay2/1
  Delay/1 -> MATLAB Function/2(u2)
  Delay2/1 -> MATLAB Function/5(old_amplitude)
  Delay1/1 -> MATLAB Function/3(u3)
  new_amplitude/1 -> MATLAB Function/4(new_amplitude)

== system opti_debug/Signal generater/signal generator1/signal generator 2/get max voltage/SIgnalForRamp_binary ==
  note: Should output 1 or -1,
      | so signal ramps UP to 1
      | or DOWN to 0.
  In1 : Inport
  Add : Sum  Inputs=+-
  Compare To Zero : simulink/Logic and Bit Operations/Compare To Zero  relop=>  OutDataTypeStr=uint8  ZeroCross=off
  Constant : Constant
  Data Type Conversion : DataTypeConversion  OutDataTypeStr=double  SaturateOnIntegerOverflow=off  RndMeth=Floor
  Gain : Gain  Gain=2
  Out1 : Outport
  wires:
  In1/1 -> Compare To Zero/1
  Compare To Zero/1 -> Data Type Conversion/1
  Gain/1 -> Add/1
  Constant/1 -> Add/2
  Add/1 -> Out1/1
  Data Type Conversion/1 -> Gain/1

== system opti_debug/Signal generater/signal generator1/signal generator 2/square root of sine wave/Subsystem1 ==
  cos wave : Inport
  new_amplitude : Inport  Port=2
  Delay : Delay  DelayLength=1  InitialCondition=0
  Delay1 : Delay  InitialCondition=[0,0]
  Delay2 : Delay  DelayLength=1  InitialCondition=0
  MATLAB Function : MATLAB Function  TreatAsAtomicUnit=on  SystemSampleTime=mdl.T_high
  output : Outport
  wires:
  cos wave/1 -> Delay1/1, Delay/1, MATLAB Function/1(u1)
  MATLAB Function/1(output) -> output/1, Delay2/1
  Delay/1 -> MATLAB Function/2(u2)
  Delay2/1 -> MATLAB Function/5(old_amplitude)
  Delay1/1 -> MATLAB Function/3(u3)
  new_amplitude/1 -> MATLAB Function/4(new_amplitude)
